simulink library "INT_InjCtl_qCo"  (R2016b)
settings: Solver=VariableStepAuto  StartTime=0.0  StopTime=10.0  RelTol=1e-3
settings Model: Creator=zhoutinglin  LastModifiedBy=zhoutinglin

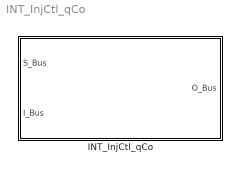
== system INT_InjCtl_qCo ==
  INT_InjCtl_qCo : Subsystem

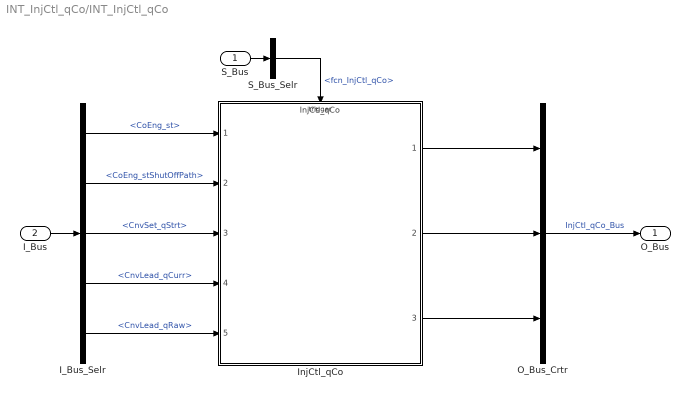
== system INT_InjCtl_qCo/INT_InjCtl_qCo ==
  S_Bus : Inport
  I_Bus : Inport  Port=2
  I_Bus_Selr : BusSelector  OutputSignals=CoEng_st,CoEng_stShutOffPath,CnvSet_qStrt,CnvLead_qCurr,CnvLead_qRaw
  InjCtl_qCo : ModelReference  ModelNameDialog=InjCtl_qCo  SimulationMode=Normal  ModelReferenceVersion=1.10  TriggerPortName=function  TriggerPortTriggerType=function-call  TriggerPortStatesWhenEnabling=held
  O_Bus_Crtr : BusCreator  Inputs=3
  S_Bus_Selr : BusSelector  OutputSignals=fcn_InjCtl_qCo
  O_Bus : Outport
  wires:
  S_Bus_Selr/1 -> InjCtl_qCo/Trigger  "<fcn_InjCtl_qCo>"
  S_Bus/1 -> S_Bus_Selr/1
  I_Bus/1 -> I_Bus_Selr/1
  I_Bus_Selr/1 -> InjCtl_qCo/1  "<CoEng_st>"
  I_Bus_Selr/2 -> InjCtl_qCo/2  "<CoEng_stShutOffPath>"
  I_Bus_Selr/3 -> InjCtl_qCo/3  "<CnvSet_qStrt>"
  I_Bus_Selr/4 -> InjCtl_qCo/4  "<CnvLead_qCurr>"
  I_Bus_Selr/5 -> InjCtl_qCo/5  "<CnvLead_qRaw>"
  O_Bus_Crtr/1 -> O_Bus/1  "InjCtl_qCo_Bus"
  InjCtl_qCo/1 -> O_Bus_Crtr/1
  InjCtl_qCo/2 -> O_Bus_Crtr/2
  InjCtl_qCo/3 -> O_Bus_Crtr/3
